simulink model "T2_critical_gain_me23b201"  (R2025a)
settings: Solver=VariableStepAuto  StartTime=0.0  StopTime=100.0  RelTol=1e-3
undefined symbols (not defined in the file or in its folder): Gm
settings Model: Creator=abhi  LastModifiedBy=abhi

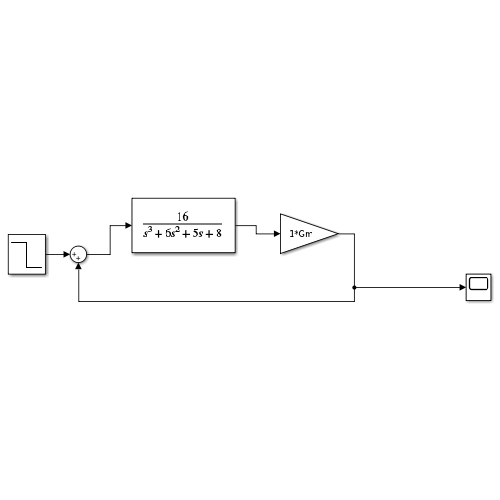
[thumbnail: Simulink's stored preview of the top-level diagram]
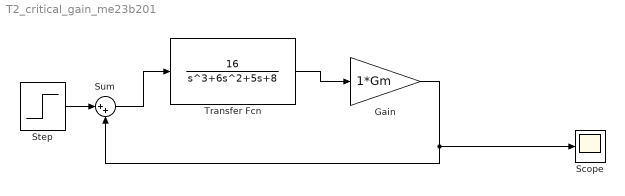
== system T2_critical_gain_me23b201 ==
  Gain : Gain  Gain=1*Gm
  Scope : Scope
      settings: ActiveDisplayYMinimum=-1.2769234497974784E+31  ActiveDisplayYMaximum=1.1492311048177308E+32
  Step : Step  Before=1  After=0  SampleTime=0
  Sum : Sum  Inputs=|++
  Transfer Fcn : TransferFcn  Numerator=[16]  Denominator=[1 6 5 8]
  wires:
  Step/1 -> Sum/1
  Sum/1 -> Transfer Fcn/1
  Transfer Fcn/1 -> Gain/1
  Gain/1 -> Sum/2, Scope/1
